simulink model "Blink_LED"  (R2024a)
settings: Solver=VariableStepAuto  StartTime=0.0  StopTime=10  RelTol=1e-3
settings Model: Creator=VICTUS  LastModifiedBy=VICTUS

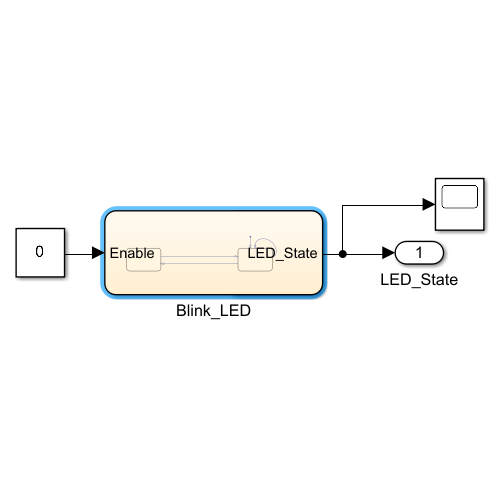
[thumbnail: Simulink's stored preview of the top-level diagram]
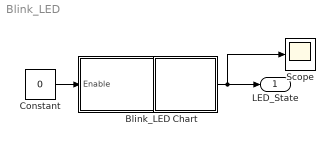
== system Blink_LED ==
  Blink_LED : Stateflow chart  TreatAsAtomicUnit=on
  Chart : Stateflow chart  TreatAsAtomicUnit=on
  Constant : Constant  Value=0
  Scope : Scope
  LED_State : Outport
  wires:
  Blink_LED/1(LED_State) -> Scope/1, LED_State/1
  Constant/1 -> Blink_LED/1(Enable)

== stateflow chart Blink_LED/Blink_LED ==
  state LED_ON
    entry:
    LED_State = 1;
  state LED_OFF
    entry:
    LED_State = 0;
  (default) -> LED_OFF
  LED_OFF -> LED_OFF [order 2] : [Enable == 0]
  LED_ON -> LED_OFF : after(1,sec)
  LED_OFF -> LED_ON [order 1] : after(1,sec)
  data: LED_State output double; Enable input

== stateflow chart Blink_LED/Chart ==
